simulink model "sim3"  (R2016b)
settings: Solver=ode4  StartTime=0.0  StopTime=t  FixedStep=0.002  RelTol=1e-3  EnableMultiTasking=on
values from neighbouring files (symbols this model uses):
  Jm = 3.9e-7    (= 3.9e-07)    [prelab4.m]
  KD = 40    [prelab4.m]
  Kg = 3.71    [prelab4.m]
  Km = 7.67e-3    (= 0.00767)    [prelab4.m]
  Kt = 7.67e-3    (= 0.00767)    [prelab4.m]
  mc = 0.94    [prelab4.m]
  r = 6.36e-3    (= 0.00636)    [prelab4.m]
  Rm = 2.6    [prelab4.m]
settings Model: Creator=ThinkPad  LastModifiedBy=Thinkpad
settings OptimizationCC: LifeSpan=inf
settings DebuggingCC: SFUnexpectedBacktrackingDiag=warning  SFNoUnconditionalDefaultTransitionDiag=warning  SFExecutionAtInitializationDiag=none
settings GRTTargetCC: TargetLangStandard=C89/C90 (ANSI)  GeneratePreprocessorConditionals=Disable all
settings ConfigComp: CovMetricSettings=dw  CovHtmlReporting=on  CovSaveCumulativeToWorkspaceVar=on  CovSaveSingleToWorkspaceVar=on  CovExternalEMLEnable=off

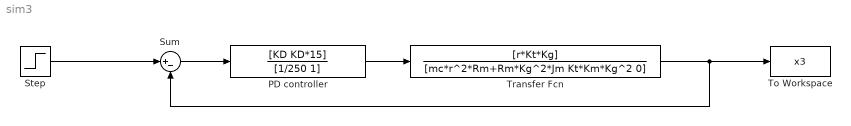
== system sim3 ==
  PD controller : TransferFcn  Numerator=[KD KD*15]  Denominator=[1/250 1]
  Step : Step  Time=0  SampleTime=0
  Sum : Sum  Inputs=|+-
  To Workspace : ToWorkspace  VariableName=x3  SaveFormat=Timeseries  SampleTime=-1
  Transfer Fcn : TransferFcn  Numerator=[r*Kt*Kg]  Denominator=[mc*r^2*Rm+Rm*Kg^2*Jm Kt*Km*Kg^2 0]
  wires:
  Step/1 -> Sum/1
  Sum/1 -> PD controller/1
  PD controller/1 -> Transfer Fcn/1
  Transfer Fcn/1 -> Sum/2, To Workspace/1
